simulink model "SerialSendReceive_5sensores"  (R2020b)
settings: Solver=FixedStepDiscrete  StartTime=0.0  StopTime=inf  FixedStep=0.01  RelTol=1e-3
libraries: arduinolib x10, simulink x4, pid_lib x2
settings Model: SimulationMode=external  ExtModeTrigDuration=2  Creator=Pablo  LastModifiedBy=manol
settings SolverCC: AutoInsertRateTranBlk=on
settings DataIOCC: ReturnWorkspaceOutputs=off
settings OptimizationCC: PassReuseOutputArgsAs=Individual arguments  MaxStackSize=64  EfficientTunableParamExpr=on
settings DebuggingCC: ParameterOverflowMsg=none  ParameterPrecisionLossMsg=none  ParameterTunabilityLossMsg=error  ArithmeticOperatorsInVariantConditions=warning
settings HardwareCC: ProdBitPerInt=16  ProdBitPerPointer=16  ProdBitPerSizeT=16  ProdBitPerPtrDiffT=16  ProdLargestAtomicFloat=None  ProdWordSize=8  ProdHWDeviceType=Atmel->AVR  UseEmbeddedCoderFeatures=off  UseSimulinkCoderFeatures=off
settings SFSimCC: SimUseLocalCustomCode=off  MATLABDynamicMemAlloc=off  CustomCodeUndefinedFunction=UseInterfaceOnly
settings RTWCC: Description=Embedded Coder  SystemTargetFile=ert.tlc  HardwareBoard=Arduino Mega 2560  TemplateMakefile=ert_default_tmf  RTWVerbose=off  RTWUseLocalCustomCode=off  Toolchain=Arduino AVR  BuildConfiguration=Faster Runs  IncludeHyperlinkInReport=on
settings CodeAppCC: ForceParamTrailComments=on  OperatorAnnotations=on  SimulinkDataObjDesc=on  SFDataObjDesc=on  MangleLength=10  InsertBlockDesc=on
settings ERTTargetCC: SupportContinuousTime=on  SupportNonInlinedSFcns=on  SupportVariableSizeSignals=on  ExtMode=on  ExtModeMexArgs='127.0.0.1' 0 17725  ERTSrcFileBannerTemplate=codertarget_code_template.cgt  ERTHdrFileBannerTemplate=codertarget_code_template.cgt  ERTDataSrcFileTemplate=codertarget_code_template.cgt  ERTDataHdrFileTemplate=codertarget_code_template.cgt

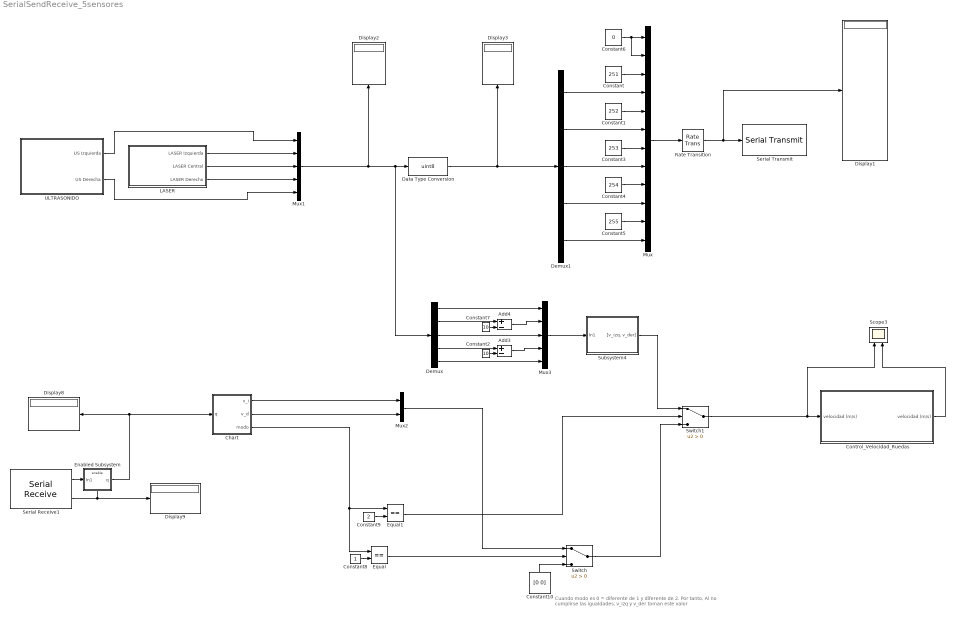
== system SerialSendReceive_5sensores ==
  note: Cuando modo es 0 = diferente de 1 y diferente de 2.
      | Por tanto, Al no cumplirse las igualdades, v_izq y v_der toman este valor
  Add3 : Sum  Inputs=+-  AccumDataTypeStr=int32  OutDataTypeStr=int32
  Add4 : Sum  Inputs=+-  AccumDataTypeStr=int32  OutDataTypeStr=int32
  Chart : Stateflow chart  TreatAsAtomicUnit=on
  Constant : Constant  Value=251  OutDataTypeStr=uint8
  Constant1 : Constant  Value=252  OutDataTypeStr=uint8
  Constant10 : Constant  Value=[0 0]
  Constant2 : Constant  Value=10
  Constant3 : Constant  Value=253  OutDataTypeStr=uint8
  Constant4 : Constant  Value=254  OutDataTypeStr=uint8
  Constant5 : Constant  Value=255  OutDataTypeStr=uint8
  Constant6 : Constant  Value=0  OutDataTypeStr=uint8
  Constant7 : Constant  Value=10
  Constant8 : Constant
  Constant9 : Constant  Value=2
  Control_Velocidad_Ruedas : Subsystem
  Data Type Conversion : DataTypeConversion  OutDataTypeStr=uint8
  Demux : Demux  Outputs=5
  Demux1 : Demux  Outputs=5
  Display{1..3,8..9} (5 alike) : Display
  Enabled Subsystem : Subsystem  TreatAsAtomicUnit=on
  Equal : RelationalOperator  Operator===  OutDataTypeStr=boolean  RndMeth=Simplest
  Equal1 : RelationalOperator  Operator===  OutDataTypeStr=boolean  RndMeth=Simplest
  LASER : Subsystem
  Mux : Mux  Inputs=12
  Mux1 : Mux  Inputs=5
  Mux2 : Mux  Inputs=2
  Mux3 : Mux  Inputs=5
  Rate Transition : RateTransition  OutPortSampleTime=1
  Scope3 : Scope  NumInputPorts=2
  Serial Receive1 : arduinolib/Serial Receive  isARMArch=off  portNumber=3  DataType=uint8  Datalength=1  SampleTime=0.01  showOutStatus=on  blockPlatform=arduino
      settings: SourceProductBaseCode=ARDUINO
  Serial Transmit : arduinolib/Serial Transmit  portNumber=3  sendmode=write  label=sensores  sendformat=Decimal  floatprecision=2  blockPlatform=arduino
  Subsystem4 : Subsystem
  Switch : Switch  Criteria=u2 > Threshold
  Switch1 : Switch  Criteria=u2 > Threshold
  "ULTRASONIDO " : Subsystem
  wires:
  Rate Transition/1 -> Display1/1, Serial Transmit/1
  Constant/1 -> Mux/3
  Constant1/1 -> Mux/5
  Constant3/1 -> Mux/7
  Constant4/1 -> Mux/9
  Constant5/1 -> Mux/11
  Mux/1 -> Rate Transition/1
  Constant6/1 -> Mux/2, Mux/1
  Data Type Conversion/1 -> Demux1/1, Display3/1
  Mux1/1 -> Data Type Conversion/1, Demux/1, Display2/1
  "ULTRASONIDO "/2(US Derecha) -> Mux1/5
  "ULTRASONIDO "/1(US Izquierda) -> Mux1/1
  Demux1/1 -> Mux/4
  Demux1/2 -> Mux/6
  Demux1/3 -> Mux/8
  Demux1/4 -> Mux/10
  Demux1/5 -> Mux/12
  LASER/1(LASER Izquierda) -> Mux1/2
  LASER/2(LASER Central) -> Mux1/3
  LASER/3(LASER Derecho) -> Mux1/4
  Serial Receive1/2 -> Display9/1, Enabled Subsystem/Enable
  Serial Receive1/1 -> Enabled Subsystem/1(In1)
  Enabled Subsystem/1(q) -> Chart/1(q), Display8/1
  Control_Velocidad_Ruedas/1(velocidad (m/s)) -> Scope3/2
  Chart/1(v_i) -> Mux2/1
  Chart/2(v_d) -> Mux2/2
  Subsystem4/1("[v_izq, v_der]") -> Switch1/1
  Equal1/1 -> Switch1/2
  Switch/1 -> Switch1/3
  Constant9/1 -> Equal1/2
  Constant10/1 -> Switch/3
  Equal/1 -> Switch/2
  Constant8/1 -> Equal/2
  Chart/3(modo) -> Equal/1, Equal1/1
  Switch1/1 -> Scope3/1, Control_Velocidad_Ruedas/1(velocidad (m/s))
  Mux2/1 -> Switch/1
  Demux/5 -> Mux3/5
  Demux/1 -> Mux3/1
  Demux/3 -> Mux3/3
  Constant2/1 -> Add3/2
  Demux/4 -> Add3/1
  Add3/1 -> Mux3/4
  Constant7/1 -> Add4/2
  Add4/1 -> Mux3/2
  Demux/2 -> Add4/1
  Mux3/1 -> Subsystem4/1(In1)

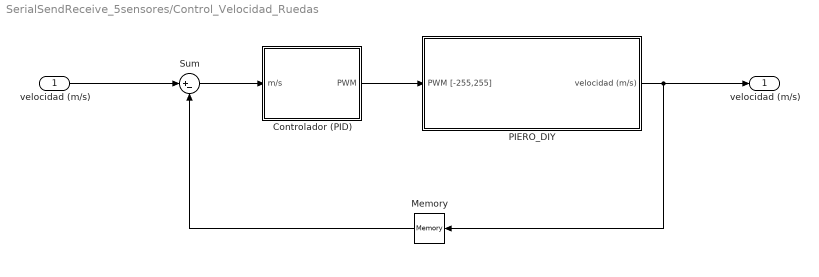
== system SerialSendReceive_5sensores/Control_Velocidad_Ruedas ==
  velocidad (m/s) : Inport
  Controlador (PID) : Subsystem
  Memory : Memory
  PIERO_DIY : Subsystem
  Sum : Sum  Inputs=|+-
  velocidad (m/s) : Outport  VectorParamsAs1DForOutWhenUnconnected=off
  wires:
  velocidad (m/s)/1 -> Sum/1
  PIERO_DIY/1(velocidad (m/s)) -> velocidad (m/s)/1, Memory/1
  Sum/1 -> Controlador (PID)/1(m/s)
  Controlador (PID)/1(PWM) -> PIERO_DIY/1(PWM [-255,255])
  Memory/1 -> Sum/2

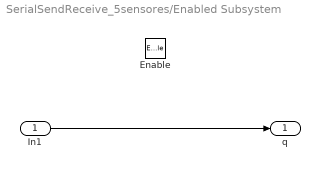
== system SerialSendReceive_5sensores/Enabled Subsystem ==
  In1 : Inport
  Enable : EnablePort
  q : Outport
  wires:
  In1/1 -> q/1

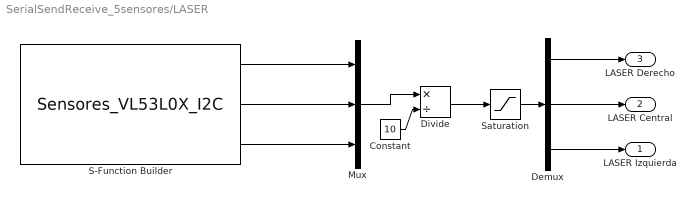
== system SerialSendReceive_5sensores/LASER ==
  Constant : Constant  Value=10
  Demux : Demux  Outputs=3
  Divide : Product  Inputs=*/
  Mux : Mux  Inputs=3
  S-Function Builder : S-Function  InitFcn=try, set_param(gcb,'FunctionName','Sensores_VL53L0X_I2C'), end  FunctionName=Sensores_VL53L0X_I2C  SFunctionModules=Sensores_VL53L0X_I2C_wrapper  SFunctionDeploymentMode=off  EnableBusSupport=off  mask(S-Function Builder){}
      mask help: Simulink:masks:SFunctionBuilder_MD
      mask init:
      | val = [[.9  0.75 0.75 1 1 .9 .9 1]',[1 1 0.75 0.75 .9 .9 1 .9]'];try , sys = get_param(gcb,'SfunBuilderFcnName');if isempty(sys), sys = get_param(gcb,'FunctionName'); end,catch, sys = get_param(gcb,'FunctionName'); end
      settings: CopyFcn=set_param(gcbh,'LinkStatus','none')  PreSaveFcn=try, set_param(gcb,'FunctionName','Sensores_VL53L0X_I2C'), end  OpenFcn=sfunctionwizard(gcbh)
      mask Display:
      | plot(val(:,1),val(:,2))
      | disp(sys)
      | port_label('output',1,'Sensor1')
      | port_label('output',2,'Sensor2')
      | port_label('output',3,'Sensor3')
  Saturation : Saturate  UpperLimit=255  LowerLimit=0
  LASER Izquierda : Outport  VectorParamsAs1DForOutWhenUnconnected=off
  LASER Central : Outport  Port=2  VectorParamsAs1DForOutWhenUnconnected=off
  LASER Derecho : Outport  Port=3  VectorParamsAs1DForOutWhenUnconnected=off
  wires:
  Mux/1 -> Divide/1
  S-Function Builder/1 -> Mux/1
  S-Function Builder/2 -> Mux/2
  S-Function Builder/3 -> Mux/3
  Demux/2 -> LASER Central/1
  Demux/1 -> LASER Derecho/1
  Demux/3 -> LASER Izquierda/1
  Divide/1 -> Saturation/1
  Saturation/1 -> Demux/1
  Constant/1 -> Divide/2

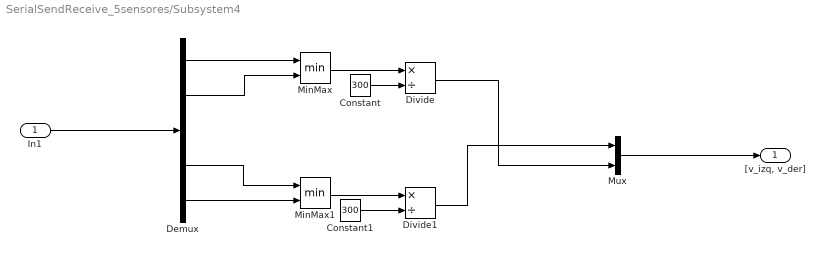
== system SerialSendReceive_5sensores/Subsystem4 ==
  In1 : Inport
  Constant : Constant  Value=300
  Constant1 : Constant  Value=300
  Demux : Demux  Outputs=5
  Divide : Product  Inputs=*/
  Divide1 : Product  Inputs=*/
  MinMax : MinMax  Inputs=2
  MinMax1 : MinMax  Inputs=2
  Mux : Mux  Inputs=2
  "[v_izq, v_der]" : Outport
  wires:
  MinMax/1 -> Divide/1
  Demux/1 -> MinMax/1
  Demux/5 -> MinMax1/2
  MinMax1/1 -> Divide1/1
  Demux/4 -> MinMax1/1
  Demux/2 -> MinMax/2
  In1/1 -> Demux/1
  Constant/1 -> Divide/2
  Constant1/1 -> Divide1/2
  Divide1/1 -> Mux/1
  Divide/1 -> Mux/2
  Mux/1 -> "[v_izq, v_der]"/1

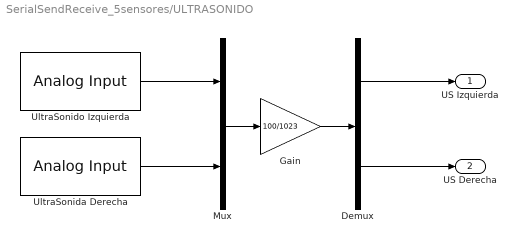
== system SerialSendReceive_5sensores/ULTRASONIDO  ==
  Demux : Demux  Outputs=2
  Gain : Gain  Gain=100/1023  OutDataTypeStr=int32
  Mux : Mux  Inputs=2
  UltraSonida Derecha : arduinolib/Analog Input  pinNumber=0  ReadResultsOnly=off  ConversionTriggerSource=Software  ExternalTriggerType=uint32( 0 )  OutputDataType=uint16  EnableConversionCompleteNotify=off  EnableOuputStatus=off  SampleTime=0.1  blockPlatform=arduino
  UltraSonido Izquierda : arduinolib/Analog Input  pinNumber=1  ReadResultsOnly=off  ConversionTriggerSource=Software  ExternalTriggerType=uint32( 0 )  OutputDataType=uint16  EnableConversionCompleteNotify=off  EnableOuputStatus=off  SampleTime=0.1  blockPlatform=arduino
  US Izquierda : Outport
  US Derecha : Outport  Port=2
  wires:
  Demux/1 -> US Izquierda/1
  Demux/2 -> US Derecha/1
  UltraSonida Derecha/1 -> Mux/2
  UltraSonido Izquierda/1 -> Mux/1
  Mux/1 -> Gain/1
  Gain/1 -> Demux/1

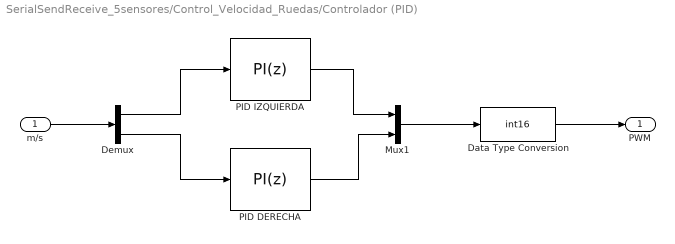
== system SerialSendReceive_5sensores/Control_Velocidad_Ruedas/Controlador (PID) ==
  m/s : Inport
  Data Type Conversion : DataTypeConversion  OutDataTypeStr=int16
  Demux : Demux  Outputs=2
  Mux1 : Mux  Inputs=2
  PID DERECHA : pid_lib/PID Controller  Controller=PI  Form=Parallel  TimeDomain=Discrete-time  UseExternalTs=off  SampleTime=0.01  IntegratorMethod=Forward Euler  FilterMethod=Forward Euler  ControllerParametersSource=internal  P=4.23623623482931  I=847.247246965862  D=0  UseFilter=on  N=100  TunerSelectOption=Transfer Function Based (PID Tuner App)  InitialConditionSource=internal  InitialConditionForIntegrator=0  InitialConditionForFilter=0  DifferentiatorICPrevScaledInput=0  ExternalReset=none  TrackingMode=off  Kt=1  LimitOutput=on  SatLimitsSource=internal  UpperSaturationLimit=255  LowerSaturationLimit=0  LinearizeAsGain=on  AntiWindupMode=none  Kb=1  POutMin=[]  POutMax=[]  IOutMin=[]  IOutMax=[]  DOutMin=[]  DOutMax=[]  NOutMin=[]  NOutMax=[]  SumOutMin=[]  SumOutMax=[]  SaturationOutMin=[]  SaturationOutMax=[]  PParamMin=[]  PParamMax=[]  IParamMin=[]  IParamMax=[]  DParamMin=[]  DParamMax=[]  NParamMin=[]  NParamMax=[]  KbParamMin=[]  KbParamMax=[]  KtParamMin=[]  KtParamMax=[]  KbOutMin=[]  KbOutMax=[]  KtOutMin=[]  KtOutMax=[]  IntegratorOutMin=[]  IntegratorOutMax=[]  FilterOutMin=[]  FilterOutMax=[]  SumI1OutMin=[]  SumI1OutMax=[]  SumI2OutMin=[]  SumI2OutMax=[]  SumI3OutMin=[]  SumI3OutMax=[]  SumI4OutMin=[]  SumI4OutMax=[]  SumDOutMin=[]  SumDOutMax=[]  DifferentiatorOutMin=[]  DifferentiatorOutMax=[]  FilterDiffOutCoefMin=[]  FilterDiffOutCoefMax=[]  ReciprocalOutMin=[]  ReciprocalOutMax=[]  SumDenOutMin=[]  SumDenOutMax=[]  SumNumOutMin=[]  SumNumOutMax=[]  DivideOutMin=[]  DivideOutMax=[]  UdiffTsProdOutMin=[]  UdiffTsProdOutMax=[]  NTsProdOutMin=[]  NTsProdOutMax=[]  UintegralTsProdOutMin=[]  UintegralTsProdOutMax=[]  UngainTsProdOutMin=[]  UngainTsProdOutMax=[]  IntegratorContinuousStateAttributes=''  IntegratorStateMustResolveToSignalObject=off  IntegratorRTWStateStorageClass=Auto  FilterContinuousStateAttributes=''  FilterStateMustResolveToSignalObject=off  FilterRTWStateStorageClass=Auto  ParallelPVariant=InternalParameters  IdealPVariant=Disabled  IVariant=InternalParameters  DVariant=Disabled  IntegratorVariant=Discrete  SatVariant=Enabled  AWVariant=Passthrough  PCopyVariant=Disabled  TRVariant=Disabled  FdbkBlocksVariant=Forward  IdealPFdbkVariant=Disabled  SatFdbkVariant=Disabled  DerivativeFilterVariant=Disabled  NVariant=Disabled  NCopyVariant=Disabled_SignalSpec  FilterICVariant=Disabled  IntegratorICVariant=InternalICs  ExternalResetVariant=Disabled  TRSumVariant=Passthrough  SumFdbkVariant=Disabled  SumVariant=Sum_PI  TsampFilterVariant=InternalTs  TsampNgainVariant=Passthrough  TsampIntegralVariant=Passthrough  ExternalSaturationOutDataTypeStr=Inherit: Same as second input
  PID IZQUIERDA : pid_lib/PID Controller  Controller=PI  Form=Parallel  TimeDomain=Discrete-time  UseExternalTs=off  SampleTime=0.01  IntegratorMethod=Forward Euler  FilterMethod=Forward Euler  ControllerParametersSource=internal  P=4.18488568996179  I=836.977137992358  D=0  UseFilter=on  N=100  TunerSelectOption=Transfer Function Based (PID Tuner App)  InitialConditionSource=internal  InitialConditionForIntegrator=0  InitialConditionForFilter=0  DifferentiatorICPrevScaledInput=0  ExternalReset=none  TrackingMode=off  Kt=1  LimitOutput=on  SatLimitsSource=internal  UpperSaturationLimit=255  LowerSaturationLimit=0  LinearizeAsGain=on  AntiWindupMode=none  Kb=1  POutMin=[]  POutMax=[]  IOutMin=[]  IOutMax=[]  DOutMin=[]  DOutMax=[]  NOutMin=[]  NOutMax=[]  SumOutMin=[]  SumOutMax=[]  SaturationOutMin=[]  SaturationOutMax=[]  PParamMin=[]  PParamMax=[]  IParamMin=[]  IParamMax=[]  DParamMin=[]  DParamMax=[]  NParamMin=[]  NParamMax=[]  KbParamMin=[]  KbParamMax=[]  KtParamMin=[]  KtParamMax=[]  KbOutMin=[]  KbOutMax=[]  KtOutMin=[]  KtOutMax=[]  IntegratorOutMin=[]  IntegratorOutMax=[]  FilterOutMin=[]  FilterOutMax=[]  SumI1OutMin=[]  SumI1OutMax=[]  SumI2OutMin=[]  SumI2OutMax=[]  SumI3OutMin=[]  SumI3OutMax=[]  SumI4OutMin=[]  SumI4OutMax=[]  SumDOutMin=[]  SumDOutMax=[]  DifferentiatorOutMin=[]  DifferentiatorOutMax=[]  FilterDiffOutCoefMin=[]  FilterDiffOutCoefMax=[]  ReciprocalOutMin=[]  ReciprocalOutMax=[]  SumDenOutMin=[]  SumDenOutMax=[]  SumNumOutMin=[]  SumNumOutMax=[]  DivideOutMin=[]  DivideOutMax=[]  UdiffTsProdOutMin=[]  UdiffTsProdOutMax=[]  NTsProdOutMin=[]  NTsProdOutMax=[]  UintegralTsProdOutMin=[]  UintegralTsProdOutMax=[]  UngainTsProdOutMin=[]  UngainTsProdOutMax=[]  IntegratorContinuousStateAttributes=''  IntegratorStateMustResolveToSignalObject=off  IntegratorRTWStateStorageClass=Auto  FilterContinuousStateAttributes=''  FilterStateMustResolveToSignalObject=off  FilterRTWStateStorageClass=Auto  ParallelPVariant=InternalParameters  IdealPVariant=Disabled  IVariant=InternalParameters  DVariant=Disabled  IntegratorVariant=Discrete  SatVariant=Enabled  AWVariant=Passthrough  PCopyVariant=Disabled  TRVariant=Disabled  FdbkBlocksVariant=Forward  IdealPFdbkVariant=Disabled  SatFdbkVariant=Disabled  DerivativeFilterVariant=Disabled  NVariant=Disabled  NCopyVariant=Disabled_SignalSpec  FilterICVariant=Disabled  IntegratorICVariant=InternalICs  ExternalResetVariant=Disabled  TRSumVariant=Passthrough  SumFdbkVariant=Disabled  SumVariant=Sum_PI  TsampFilterVariant=InternalTs  TsampNgainVariant=Passthrough  TsampIntegralVariant=Passthrough  ExternalSaturationOutDataTypeStr=Inherit: Same as second input
  PWM : Outport  VectorParamsAs1DForOutWhenUnconnected=off
  wires:
  Demux/1 -> PID IZQUIERDA/1
  Mux1/1 -> Data Type Conversion/1
  PID DERECHA/1 -> Mux1/2
  Demux/2 -> PID DERECHA/1
  m/s/1 -> Demux/1
  PID IZQUIERDA/1 -> Mux1/1
  Data Type Conversion/1 -> PWM/1

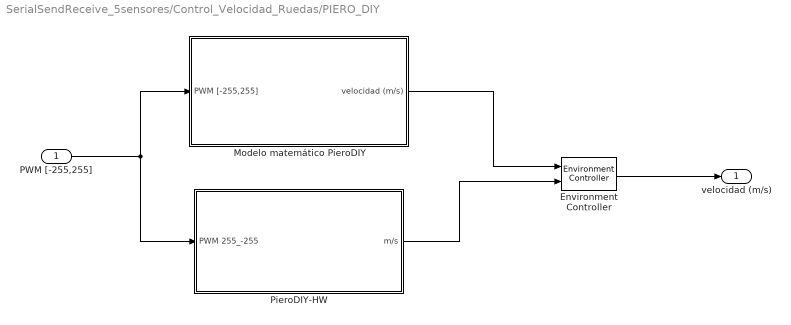
== system SerialSendReceive_5sensores/Control_Velocidad_Ruedas/PIERO_DIY ==
  PWM [-255,255] : Inport
  Environment Controller : simulink/Signal Routing/Environment Controller
      settings: SourceProductBaseCode=SL
  Modelo matemático PieroDIY : Subsystem
  PieroDIY-HW : Subsystem
  velocidad (m/s) : Outport  VectorParamsAs1DForOutWhenUnconnected=off
  wires:
  Environment Controller/1 -> velocidad (m/s)/1
  PWM [-255,255]/1 -> PieroDIY-HW/1(PWM 255_-255), Modelo matemático PieroDIY/1(PWM [-255,255])
  PieroDIY-HW/1(m/s) -> Environment Controller/2
  Modelo matemático PieroDIY/1(velocidad (m/s)) -> Environment Controller/1

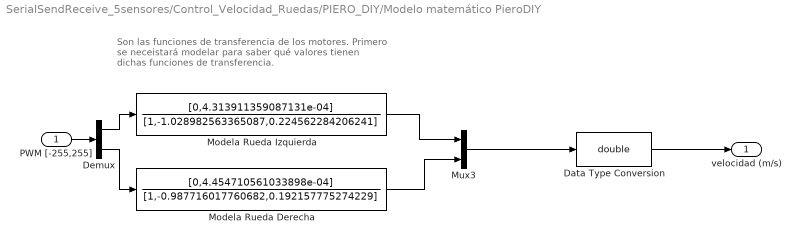
== system SerialSendReceive_5sensores/Control_Velocidad_Ruedas/PIERO_DIY/Modelo matemático PieroDIY ==
  note: Son las funciones de transferencia de los motores.
      | Primero se neceistará modelar para saber qué valores
      | tienen dichas funciones de transferencia.
  PWM [-255,255] : Inport
  Data Type Conversion : DataTypeConversion  OutDataTypeStr=double
  Demux : Demux  Outputs=2
  Modela Rueda Derecha : DiscreteFilter  Numerator=[0,4.454710561033898e-04]  Denominator=[1,-0.987716017760682,0.192157775274229]
  "Modela Rueda Izquierda " : DiscreteFilter  Numerator=[0,4.313911359087131e-04]  Denominator=[1,-1.028982563365087,0.224562284206241]
  Mux3 : Mux  Inputs=2
  velocidad (m/s) : Outport  VectorParamsAs1DForOutWhenUnconnected=off
  wires:
  Demux/2 -> Modela Rueda Derecha/1
  Data Type Conversion/1 -> velocidad (m/s)/1
  Demux/1 -> "Modela Rueda Izquierda "/1
  Mux3/1 -> Data Type Conversion/1
  Modela Rueda Derecha/1 -> Mux3/2
  PWM [-255,255]/1 -> Demux/1
  "Modela Rueda Izquierda "/1 -> Mux3/1

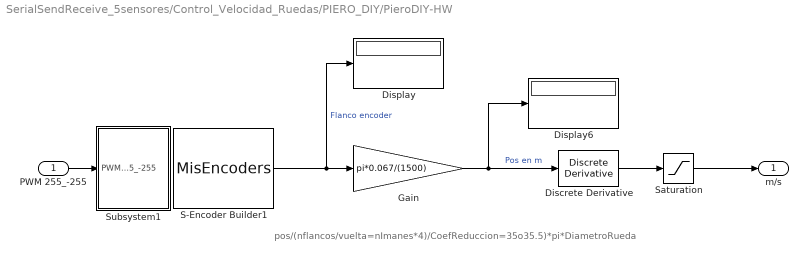
== system SerialSendReceive_5sensores/Control_Velocidad_Ruedas/PIERO_DIY/PieroDIY-HW ==
  note: pos/(nflancos/vuelta=nImanes*4)/CoefReduccion=35o35.5)*pi*DiametroRueda
  PWM 255_-255 : Inport
  Discrete Derivative : simulink/Discrete/Discrete Derivative  gainval=1.0  ICPrevScaledInput=0.0  OutMin=[]  OutMax=[]  OutDataType=fixdt(1, 16)  OutScaling=2^-10  DoSatur=off
  Display : Display
  Display6 : Display
  Gain : Gain  Gain=pi*0.067/(1500)
  S-Encoder Builder1 : S-Function  FunctionName=MisEncoders  Parameters=uint8(18),uint8(19),int8(1),uint8(2),uint8(3),uint8(0)  SFunctionModules=MisEncoders_wrapper  SFunctionDeploymentMode=off  EnableBusSupport=off  mask(S-Function Builder){}
      mask help: Simulink:masks:SFunctionBuilder_MD
      mask init: same as SerialSendReceive_5sensores/LASER/S-Function Builder
      settings: CopyFcn=set_param(gcbh,'LinkStatus','none')  PreSaveFcn=try, set_param(gcb,'FunctionName','MisEncoders'), end  OpenFcn=sfunctionwizard(gcbh)
      mask Display:
      | plot(val(:,1),val(:,2))
      | disp(sys)
      | port_label('output',1,'pos')
  Saturation : Saturate  UpperLimit=0.6  LowerLimit=-0.6
  Subsystem1 : Subsystem
  m/s : Outport  VectorParamsAs1DForOutWhenUnconnected=off
  wires:
  Discrete Derivative/1 -> Saturation/1
  Saturation/1 -> m/s/1
  PWM 255_-255/1 -> Subsystem1/1(PWM 255_-255)
  Gain/1 -> Display6/1, Discrete Derivative/1  "Pos en m"
  S-Encoder Builder1/1 -> Display/1, Gain/1  "Flanco encoder"

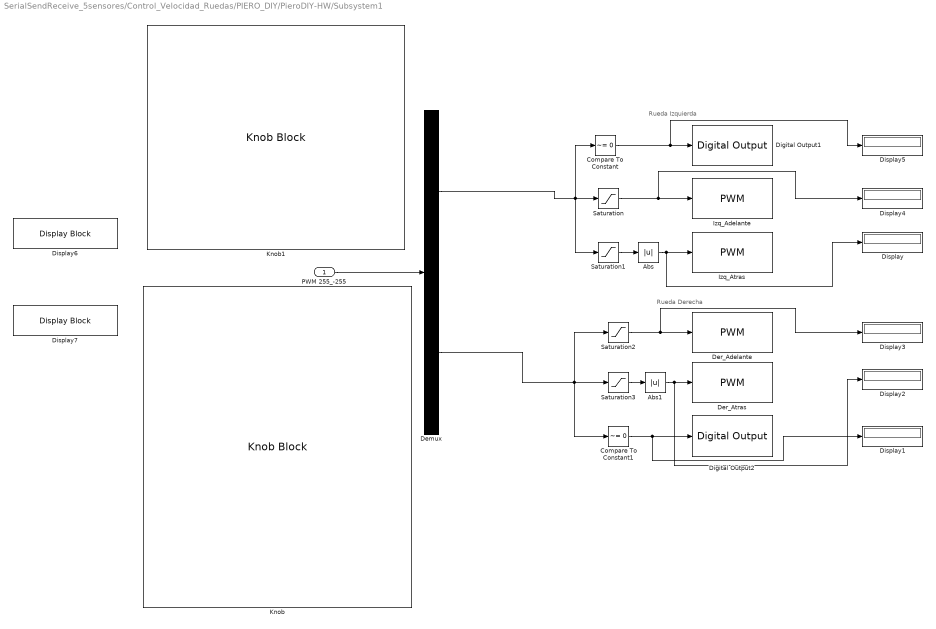
== system SerialSendReceive_5sensores/Control_Velocidad_Ruedas/PIERO_DIY/PieroDIY-HW/Subsystem1 ==
  note: Rueda Derecha
  note: Rueda Izquierda
  PWM 255_-255 : Inport
  Abs : Abs  OutDataTypeStr=uint8
  Abs1 : Abs  OutDataTypeStr=uint8
  Compare To Constant : simulink/Logic and Bit Operations/Compare To Constant  relop=~=  const=0  OutDataTypeStr=boolean
  Compare To Constant1 : simulink/Logic and Bit Operations/Compare To Constant  relop=~=  const=0  OutDataTypeStr=boolean
  Demux : Demux  Outputs=2
  Der_Adelante : arduinolib/PWM  pinNumber=8  frequencyType=Default  desiredFrequency=490.2  achievableFrequency=490.2
  Der_Atras : arduinolib/PWM  pinNumber=9  frequencyType=Default  desiredFrequency=490.2  achievableFrequency=490.2
  Digital Output1 : arduinolib/Digital Output  pinNumber=5  Direction=output  blockPlatform=arduino
  Digital Output2 : arduinolib/Digital Output  pinNumber=10  Direction=output  blockPlatform=arduino
  Display{,1..5} (6 alike) : Display
  Display6 : DisplayBlock  LabelPosition=Hide
  Display7 : DisplayBlock  LabelPosition=Hide
  Izq_Adelante : arduinolib/PWM  pinNumber=6  frequencyType=Default  desiredFrequency=490.2  achievableFrequency=490.2
  Izq_Atras : arduinolib/PWM  pinNumber=7  frequencyType=Default  desiredFrequency=490.2  achievableFrequency=490.2
  Knob : KnobBlock
  Knob1 : KnobBlock
  Saturation : Saturate  UpperLimit=255  LowerLimit=0
  Saturation1 : Saturate  UpperLimit=0  LowerLimit=-255
  Saturation2 : Saturate  UpperLimit=255  LowerLimit=0
  Saturation3 : Saturate  UpperLimit=0  LowerLimit=-255
  wires:
  Saturation/1 -> Display4/1, Izq_Adelante/1
  Compare To Constant/1 -> Display5/1, Digital Output1/1
  Saturation1/1 -> Abs/1
  PWM 255_-255/1 -> Demux/1
  Demux/1 -> Saturation1/1, Compare To Constant/1, Saturation/1
  Abs/1 -> Display/1, Izq_Atras/1
  Saturation3/1 -> Abs1/1
  Demux/2 -> Compare To Constant1/1, Saturation2/1, Saturation3/1
  Compare To Constant1/1 -> Display1/1, Digital Output2/1
  Abs1/1 -> Display2/1, Der_Atras/1
  Saturation2/1 -> Display3/1, Der_Adelante/1

== stateflow chart SerialSendReceive_5sensores/Chart ==
  state nada
    v_i=0;
    v_d=0;
    modo=0;
  state espera1
  state Evita_obs
    entry:
    modo=2;
  state Primera_etiqueta_X1
  state espera
    entry:
    modo=1;
  state Derecha
    entry:
    if(v_d<=0.4 & v_d>=-0.2)
    v_i=v_i+0.05;
    v_d=v_d-0.02;
    end;
  state Izquierda
    entry:
    if(v_i<=0.4 & v_d>=-0.2)
    v_d=v_d+0.05;
    v_i=v_i-0.02;
    end;
  state Primera_etiqueta_X
  state Atras
    entry:
    if(v_d>=-0.2 & v_i>=-0.2)
    v_d=v_d-0.05;
    v_i=v_i-0.05;
    end;
  state Adelante
    entry:
    if(v_i<=0.4 & v_d<=0.4)
    v_i=v_i+0.05;
    v_d=v_d+0.05;
    end;
  state Parar
    entry:
    v_i=0;
    v_d=0;
  (default) -> nada
  Primera_etiqueta_X -> nada [order 2] : [q==82]
  Primera_etiqueta_X1 -> nada [order 3] : [q==82]
  nada -> espera1
  espera1 -> Primera_etiqueta_X1 : [q==88]
  Primera_etiqueta_X1 -> Evita_obs [order 2] : [q==69]
  Evita_obs -> Primera_etiqueta_X1 : [q==88]
  Primera_etiqueta_X1 -> espera [order 1] : [q==77]
  Derecha -> espera
  Izquierda -> espera
  Parar -> espera
  Atras -> espera
  Adelante -> espera
  Primera_etiqueta_X -> espera [order 7] : [q==77]
  espera -> Primera_etiqueta_X : [q==88]
  Primera_etiqueta_X -> Derecha [order 3] : [q==68]
  Primera_etiqueta_X -> Izquierda [order 1] : [q==65]
  Primera_etiqueta_X -> Atras [order 5] : [q==83]
  Primera_etiqueta_X -> Adelante [order 4] : [q==87]
  Primera_etiqueta_X -> Parar [order 6] : [q==32]
  data: v_i output; q input; v_d output; modo output
